simulink model "System_model_PID_attempt_01"  (R2020b)
settings: Solver=FixedStepAuto  StartTime=0.0  StopTime=2  FixedStep=0.001  RelTol=1e-3
settings Model: Creator=Viibrem  LastModifiedBy=Viibrem

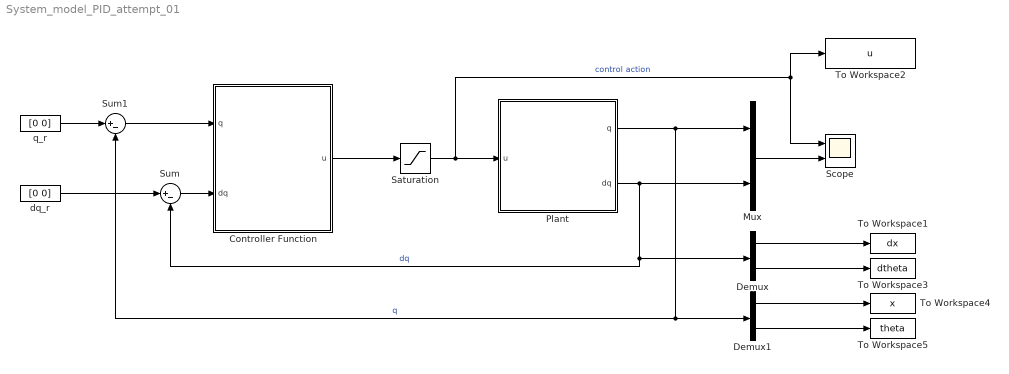
== system System_model_PID_attempt_01 ==
  Controller Function : MATLAB Function  TreatAsAtomicUnit=on
  Demux : Demux  Outputs=2
  Demux1 : Demux  Outputs=2
  Mux : Mux  Inputs=2
  Plant : Subsystem
  Saturation : Saturate  UpperLimit=3.3  LowerLimit=-3.3
  Scope : Scope  NumInputPorts=2
  Sum : Sum  Inputs=|+-
  Sum1 : Sum  Inputs=|+-
  To Workspace1 : ToWorkspace  VariableName=dx  SaveFormat=Timeseries  SampleTime=-1
  To Workspace2 : ToWorkspace  VariableName=u  SaveFormat=Timeseries  SampleTime=-1
  To Workspace3 : ToWorkspace  VariableName=dtheta  SaveFormat=Timeseries  SampleTime=-1
  To Workspace4 : ToWorkspace  VariableName=x  SaveFormat=Timeseries  SampleTime=-1
  To Workspace5 : ToWorkspace  VariableName=theta  SaveFormat=Timeseries  SampleTime=-1
  dq_r : Constant  Value=[0 0]
  q_r : Constant  Value=[0 0]
  wires:
  Plant/2(dq) -> Demux/1, Sum/2, Mux/2  "dq"
  Plant/1(q) -> Mux/1, Demux1/1, Sum1/2  "q"
  Mux/1 -> Scope/2
  dq_r/1 -> Sum/1
  q_r/1 -> Sum1/1
  Saturation/1 -> To Workspace2/1, Scope/1, Plant/1(u)  "control action"
  Demux/1 -> To Workspace1/1
  Demux/2 -> To Workspace3/1
  Demux1/2 -> To Workspace5/1
  Demux1/1 -> To Workspace4/1
  Sum1/1 -> Controller Function/1(q)
  Controller Function/1(u) -> Saturation/1
  Sum/1 -> Controller Function/2(dq)

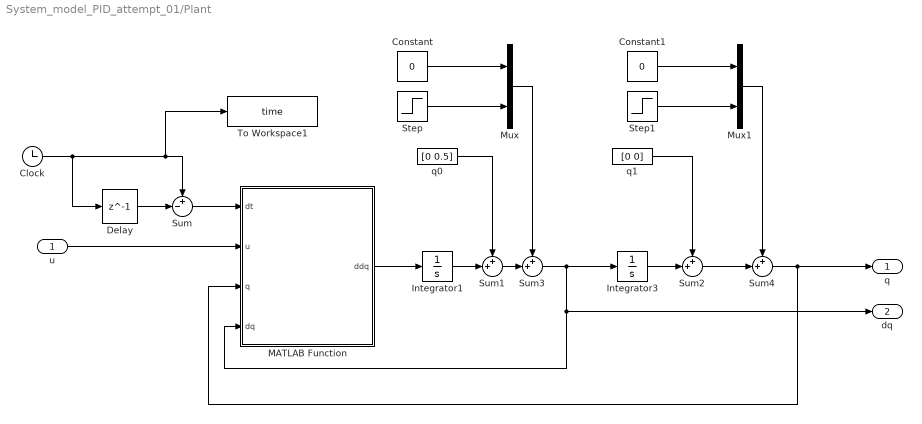
== system System_model_PID_attempt_01/Plant ==
  u : Inport
  Clock : Clock
  Constant : Constant  Value=0
  Constant1 : Constant  Value=0
  Delay : Delay  DelayLength=1  InitialCondition=0
  Integrator1 : Integrator
  Integrator3 : Integrator
  MATLAB Function : MATLAB Function  TreatAsAtomicUnit=on
  Mux : Mux  Inputs=2
  Mux1 : Mux  Inputs=2
  Step : Step  Time=0.2  After=0  SampleTime=0
  Step1 : Step  Time=0.2  After=0  SampleTime=0
  Sum : Sum  Inputs=+-|
  Sum{1..4} (4 alike) : Sum  Inputs=++|
  To Workspace1 : ToWorkspace  VariableName=time  SaveFormat=Timeseries  SampleTime=-1
  q0 : Constant  Value=[0 0.5]
  q1 : Constant  Value=[0 0]
  q : Outport
  dq : Outport  Port=2
  wires:
  Clock/1 -> To Workspace1/1, Sum/1, Delay/1
  Sum/1 -> MATLAB Function/1(dt)
  Delay/1 -> Sum/2
  MATLAB Function/1(ddq) -> Integrator1/1
  u/1 -> MATLAB Function/2(u)
  Integrator1/1 -> Sum1/2
  q0/1 -> Sum1/1
  Integrator3/1 -> Sum2/2
  q1/1 -> Sum2/1
  Sum1/1 -> Sum3/2
  Sum3/1 -> Integrator3/1, dq/1, MATLAB Function/4(dq)
  Mux/1 -> Sum3/1
  Step/1 -> Mux/2
  Constant/1 -> Mux/1
  Step1/1 -> Mux1/2
  Mux1/1 -> Sum4/1
  Constant1/1 -> Mux1/1
  Sum2/1 -> Sum4/2
  Sum4/1 -> MATLAB Function/3(q), q/1

== matlab function System_model_PID_attempt_01/Controller Function ==
  data: q input; u output; dq input
function u = fcn(q, dq)

%K = [0 0 -600 -4.7];
K = [0 0 -80 -2.5];
% K = [0 0 -100 0];
% K = [-3.1623   -0.0374  -64.2745  -11.3235];

u = K*[q(1);dq(1);q(2);dq(2)];

== matlab function System_model_PID_attempt_01/Plant/MATLAB Function ==
  data: ddq output; dt input; u input; q input; dq input
function ddq = fcn(dt, u, q, dq)

ddtheta = -0.112*dq(2) + 90.25*q(2) - 4.06*u;

ddx = -20*dq(1)+2.2*u;

ddq = [ddx,ddtheta];
